simulink model "ayrikModel"  (R2022b)
settings: Solver=FixedStepAuto  StartTime=0.0  StopTime=10.0  FixedStep=0.1  RelTol=1e-3
InitFcn:
  | ayrikModel
values from neighbouring files (symbols this model uses):
  constants = [fx_now ... (first row only)    [MST_Ayrik.m]    (also in ayrikHesaplar.m)
settings Model: Creator=aysen  LastModifiedBy=lenovo

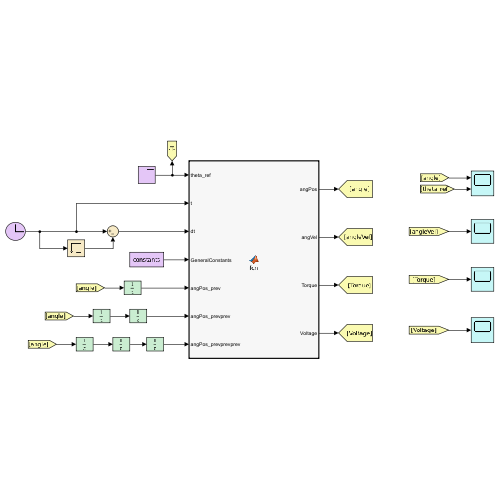
[thumbnail: Simulink's stored preview of the top-level diagram]
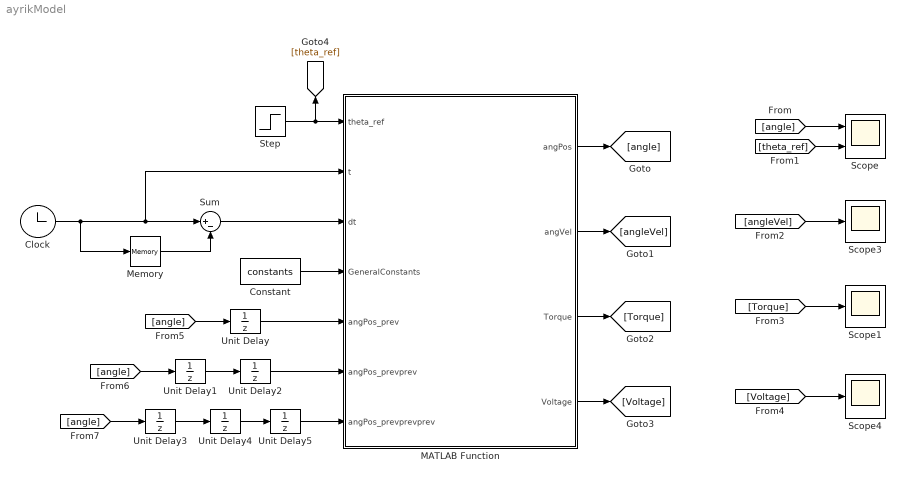
== system ayrikModel ==
  Clock : Clock
  Constant : Constant  Value=constants
  MATLAB Function : MATLAB Function  TreatAsAtomicUnit=on
  Memory : Memory
  Scope : Scope  NumInputPorts=2
  Scope1 : Scope
  Scope3 : Scope
  Scope4 : Scope
  Step : Step  After=10  SampleTime=0
  Sum : Sum  Inputs=|+-
  Unit Delay{,1..5} (6 alike) : UnitDelay  SampleTime=-1  HasFrameUpgradeWarning=on
  wires:
  Clock/1 -> MATLAB Function/2(t), Sum/1, Memory/1
  Memory/1 -> Sum/2
  Sum/1 -> MATLAB Function/3(dt)
  Constant/1 -> MATLAB Function/4(GeneralConstants)
  Step/1 -> MATLAB Function/1(theta_ref), [theta_ref]
  MATLAB Function/1(angPos) -> [angle]
  MATLAB Function/2(angVel) -> [angleVel]
  MATLAB Function/3(Torque) -> [Torque]
  MATLAB Function/4(Voltage) -> [Voltage]
  [angle] -> Scope/1
  [theta_ref] -> Scope/2
  [angleVel] -> Scope3/1
  [Torque] -> Scope1/1
  [angle] -> Unit Delay/1
  Unit Delay/1 -> MATLAB Function/5(angPos_prev)
  [angle] -> Unit Delay1/1
  Unit Delay1/1 -> Unit Delay2/1
  Unit Delay2/1 -> MATLAB Function/6(angPos_prevprev)
  Unit Delay4/1 -> Unit Delay5/1
  Unit Delay5/1 -> MATLAB Function/7(angPos_prevprevprev)
  Unit Delay3/1 -> Unit Delay4/1
  [angle] -> Unit Delay3/1
  [Voltage] -> Scope4/1

== matlab function ayrikModel/MATLAB Function ==
  data: theta_ref input size=1; angPos output size=1; angVel output; t input size=1; dt input; GeneralConstants input; Torque output size=1; angPos_prev input size=1; Voltage output; angPos_prevprev input; angPos_prevprevprev input
function [angPos, angVel, Torque, Voltage] = fcn(theta_ref,t, dt, GeneralConstants, angPos_prev,angPos_prevprev, angPos_prevprevprev)

fx_now = GeneralConstants(1,1);
fx_pre = GeneralConstants(2,1);
fx_fut = GeneralConstants(3,1);
h_fut_2 = GeneralConstants(4, 1);% eylemsizlik hesaplari
h_fut = GeneralConstants(5, 1);
h_now = GeneralConstants(6, 1);
h_pre = GeneralConstants(7, 1);
x_0 = GeneralConstants(8,1);
x_0_dot = GeneralConstants(9, 1);
%N1 = GeneralConstants(7, 1);
%N2 = GeneralConstants(8, 1);
%N3 = GeneralConstants(9, 1);

Ae = 0.5;

error = theta_ref - angPos_prev;
C1 = theta_ref - (((angPos_prev * fx_now) + (angPos_prevprev * fx_pre)) / fx_fut);

if (t == 0)
    angPos = x_0;
    Voltage = 0;
    angVel = 0;
    Torque = 0;

elseif (t == dt)
    Torque = fx_fut * (C1 - (Ae * error));
    Voltage = 0;
    angPos = x_0 + x_0_dot * dt;
    angVel = x_0_dot;

else
    Torque = fx_fut * (C1 - (Ae * error));
    angPos = (angPos_prev * fx_now + angPos_prevprev * fx_pre + Torque) / fx_fut;
    angVel = (angPos - angPos_prevprev) / (2 * dt);
    Torque = Torque * 1000;
    Voltage = (h_fut_2 * angPos) + (h_fut * angPos_prev) + ...
        (h_now * angPos_prevprev) + (h_pre * angPos_prevprevprev);
end
